simulink model "receive_2bytes_R2024b"  (R2024b)
settings: Solver=FixedStepDiscrete  StartTime=0.0  StopTime=inf  FixedStep=0.005  RelTol=1e-3  EnableMultiTasking=on
undefined symbols (not defined in the file or in its folder): b570118e, BLE_Receive, c544, df2f, eff837991f54, fce70352, receive_2bytes
libraries: arduinolib x1, svdutilitieslib x1
settings Model: ExtModeTrigDuration=2  Creator=kawata  LastModifiedBy=kawata
settings SolverCC: AutoInsertRateTranBlk=on
settings DataIOCC: ReturnWorkspaceOutputs=off
settings OptimizationCC: EnhancedBackFolding=on  PassReuseOutputArgsThreshold=0  MaxStackSize=64  OptimizeBlockOrder=speed  DifferentSizesBufferReuse=on  OptimizationCustomize=off
settings DebuggingCC: ParameterTunabilityLossMsg=error
settings HardwareCC: ProdBitPerPointer=32  ProdBitPerSizeT=32  ProdBitPerPtrDiffT=32  ProdLargestAtomicInteger=Long  ProdLargestAtomicFloat=Double  ProdWordSize=32  ProdHWDeviceType=ARM Compatible->ARM Cortex  UseEmbeddedCoderFeatures=off  UseSimulinkCoderFeatures=off
settings SFSimCC: MATLABDynamicMemAlloc=off
settings RTWCC: Description=Embedded Coder  SystemTargetFile=ert.tlc  HardwareBoard=ESP32-WROOM(Arduino Compatible)  TLCOptions="-aInlineSetEventsForThisBaseRateFcn=TLC_FALSE -aSuppressMultiTaskScheduler=TLC_FALSE  -aRateBasedStepFcn=0"  TemplateMakefile=ert_default_tmf  Toolchain=ESP32  BuildConfiguration=Faster Runs
settings CodeAppCC: ForceParamTrailComments=on  OperatorAnnotations=on
settings ERTTargetCC: ERTCustomFileBanners=off  SupportContinuousTime=on  SupportNonInlinedSFcns=on  RemoveResetFunc=off  SupportVariableSizeSignals=on  ModelStepFunctionPrototypeControlCompliant=off  ExtModeTransport=3  ExtModeStaticAlloc=on  ExtModeAutomaticAllocSize=off  ExtModeStaticAllocSize=65536  ExtModeMexFile=ext_xcp  ExtModeIntrfLevel=Level2 - Open  InlinedParameterPlacement=Hierarchical  DynamicArrayContainerType=coder::array

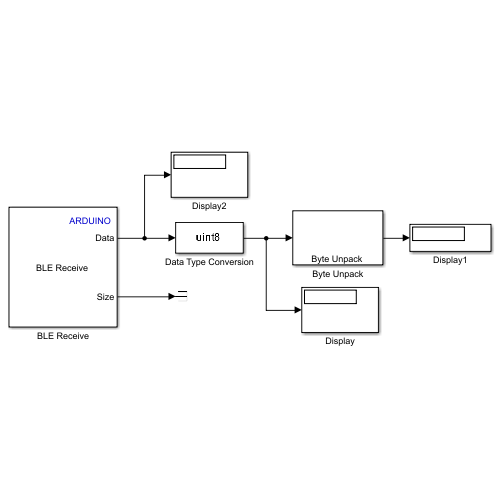
[thumbnail: Simulink's stored preview of the top-level diagram]
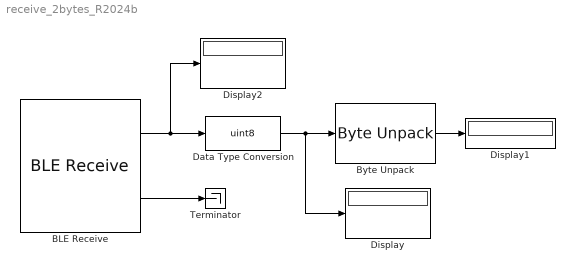
== system receive_2bytes_R2024b ==
  BLE Receive : arduinolib/BLE Receive  DeviceMode=Peripheral (Server)  BluetoothAddress=""  CharUUID=""  ServiceUUID=""  device=No Devices  character=No Characteristics  CustomService=on  ServiceName=Generic Access  CharacteristicName=Device Name  CustomServiceUUID=fce70352-c544-48f4-9760-7568263b7922  CustomCharUUID=b570118e-df2f-4545-9cf9-eff837991f54  DataSize=2  SampleTime=0.1  charseruuid=<empty>  seruuid=00001810-0000-1000-8000-00805f9b34fb  PeripheralService=00001800-0000-1000-8000-00805f9b34fb  PeripheralCharacteristic=00002a00-0000-1000-8000-00805f9b34fb  chruuid=00002a00-0000-1000-8000-00805f9b34fb  BLEId=receive_2bytes/BLE_Receive  Devicename=""  IsCustomService=0
      settings: SourceProductName=Common
  Byte Unpack : svdutilitieslib/Byte Unpack  dimensions={[1]}  datatypes={ 'int16' }  byteAlign=1  blockPlatform=arduinoert
  Data Type Conversion : DataTypeConversion  OutDataTypeStr=uint8  SaturateOnIntegerOverflow=off  RndMeth=Floor
  Display : Display
  Display1 : Display
  Display2 : Display
  Terminator : Terminator
  wires:
  BLE Receive/2 -> Terminator/1
  BLE Receive/1 -> Display2/1, Data Type Conversion/1
  Data Type Conversion/1 -> Byte Unpack/1, Display/1
  Byte Unpack/1 -> Display1/1
